simulink library "Rfm2g_syncRecv"  (Simulink 7.8)
settings: Solver=ode5  SolverMode=SingleTasking  StartTime=0.0  StopTime=Inf  FixedStep=0.001  RelTol=1e-3
settings Model: Creator=pc  LastModifiedBy=pc

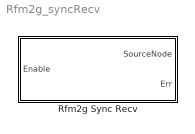
== system Rfm2g_syncRecv ==
  Rfm2g Sync Recv : Subsystem  mask(RFM2G sync recv){nodeid=0, eventtype=RFM2GEVENT_INTR1, rev0=10, rev1=0}
      mask prompts: nodeid "Node ID"; eventtype "The Sync Type of Recv"; rev0 "Timeout wait sync (ms)"
      mask help:
      | 此模块用于接收同步中断
      |
      | Node ID
      | 需要同步的节点号
      |
      | The Sync Type of Recv
      | 等待接收同步信号类型
      |
      | Timeout wait sync (ms)
      | 等待同步信号的时间阈值，必须小于等于步长值， 如给值 10 ，则在 10 内没有接收到
      | 同步信号时，Err 将返回 -1
      |
      | Enable
      | 给值 1 使能接收同步
      | SourceNode
      | 收到的同步信号的源节点号
      | Err
      | 返回 0：接收成功
      | 返回 -1：超时
      | 返回其他 ：失败
      mask init:
      | d=sprintf('Sync Recv\nNode ID %d',nodeid);
      mask StyleString: edit,popup(RFM2GEVENT_INTR1|RFM2GEVENT_INTR2|RFM2GEVENT_INTR3|RFM2GEVENT_INTR4|RFM2GEVENT_RESET),edit,edit
      mask Display: disp(d);

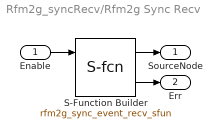
== system Rfm2g_syncRecv/Rfm2g Sync Recv ==
  Enable : Inport
  S-Function Builder : S-Function  InitFcn=try, set_param(gcb,'FunctionName','rfm2g_sync_event_recv_sfun'), end  FunctionName=rfm2g_sync_event_recv_sfun  Parameters=nodeid,eventtype,rev0,rev1  WizardData=DataTag0  EnableBusSupport=off  mask(S-Function Builder){}
      mask help: Simulink:masks:SFunctionBuilder_MD
      mask init:
      | val = [[.9  0.75 0.75 1 1 .9 .9 1]',[1 1 0.75 0.75 .9 .9 1 .9]'];try , sys = get_param(gcb,'SfunBuilderFcnName');if isempty(sys), sys = get_param(gcb,'FunctionName'); end,catch, sys = get_param(gcb,'FunctionName'); end
      settings: CopyFcn=set_param(gcbh,'LinkStatus','none')  PreSaveFcn=try, set_param(gcb,'FunctionName','rfm2g_sync_event_recv_sfun'), end  OpenFcn=sfunctionwizard(gcbh)
      mask Display: plot(val(:,1),val(:,2)),disp(sys), port_label('input',1,'u0'), port_label('input',2,'u1'), port_label('output',1,'y0'), port_label('output',2,'y1')
  SourceNode : Outport
  Err : Outport  Port=2
  wires:
  S-Function Builder/2 -> Err/1
  S-Function Builder/1 -> SourceNode/1
  Enable/1 -> S-Function Builder/1
